simulink model "AngleToPWM"  (R2018b)
settings: Solver=VariableStepAuto  StartTime=0.0  StopTime=2000  RelTol=1e-3
libraries: hdlsllib x1
settings Model: Creator=wachala.j  LastModifiedBy=vttre
settings SFSimCC: SimUseLocalCustomCode=off
settings RTWCC: RTWUseLocalCustomCode=off
settings CodeAppCC: StateflowObjectComments=on

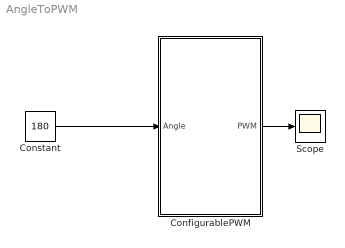
== system AngleToPWM ==
  ConfigurablePWM : Subsystem
  Constant : Constant  Value=180  OutDataTypeStr=uint8
  Scope : Scope
  wires:
  Constant/1 -> ConfigurablePWM/1(Angle)
  ConfigurablePWM/1(PWM) -> Scope/1

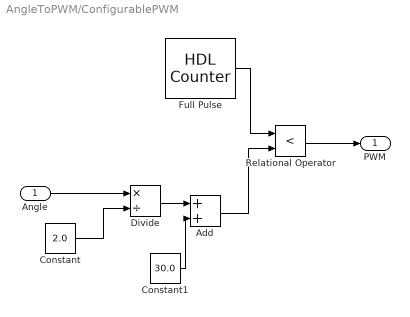
== system AngleToPWM/ConfigurablePWM ==
  Angle : Inport  OutDataTypeStr=uint8
  Add : Sum
  Constant : Constant  Value=2.0  OutDataTypeStr=uint8
  Constant1 : Constant  Value=30.0  OutDataTypeStr=uint8
  Divide : Product  Inputs=*/
  Full Pulse : hdlsllib/Sources/HDL Counter  CountType=Count limited  CountInit=0  CountStep=1  CountMax=1000  CountFromType=Initial value  CountFrom=0  CountResetPort=off  CountLoadPort=off  CountEnbPort=off  CountDirPort=off  CountDataType=Unsigned  CountWordLen=32  CountFracLen=0  CountSampTime=1
      settings: SourceProductBaseCode=HD
  Relational Operator : RelationalOperator  Operator=<  OutDataTypeStr=boolean  RndMeth=Simplest
  PWM : Outport
  wires:
  Relational Operator/1 -> PWM/1
  Full Pulse/1 -> Relational Operator/1
  Angle/1 -> Divide/1
  Constant/1 -> Divide/2
  Divide/1 -> Add/1
  Constant1/1 -> Add/2
  Add/1 -> Relational Operator/2
